simulink model "chap1_7"  (Simulink 6.3)
settings: Solver=ode4  StartTime=0.0  StopTime=1.0  RelTol=1e-3
undefined symbols (not defined in the file or in its folder): chap1_7ctrl
settings Model: LastModifiedBy=Administrator  ExtModeTrigMode=oneshot  ExtModeArmWhenConnect=off  StrictBusMsg=None
settings DataIOCC: Decimation=100  LimitDataPoints=off  SaveOutput=off  SaveTime=off
settings OptimizationCC: BlockReduction=off  BooleanDataType=off
settings DebuggingCC: SolverPrmCheckMsg=none
settings HardwareCC: TargetUnknown=on

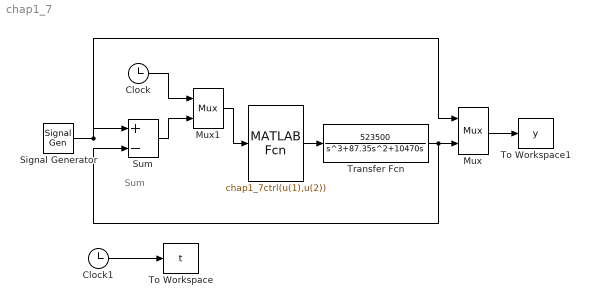
== system chap1_7 ==
  note: Sum
  "    " : MATLABFcn  MATLABFcn=chap1_7ctrl(u(1),u(2))
  Clock : Clock
      settings: Decimation=10
  Clock1 : Clock
      settings: Decimation=10
  Mux : Mux  Inputs=2
  Mux1 : Mux  Inputs=2
  Signal Generator : SignalGenerator  Amplitude=0.05
  Sum : Sum  Inputs=|+-  SaturateOnIntegerOverflow=on  InputSameDT=on
  To Workspace : ToWorkspace  VariableName=t  SampleTime=-1  SaveFormat=Array
  To Workspace1 : ToWorkspace  VariableName=y  SampleTime=-1  SaveFormat=Array
  Transfer Fcn : TransferFcn  Numerator=[523500]  Denominator=[1 87.35 10470 0]
  wires:
  Mux/1 -> To Workspace1/1
  Transfer Fcn/1 -> Sum/2, Mux/2
  Signal Generator/1 -> Sum/1, Mux/1
  Clock/1 -> Mux1/1
  Sum/1 -> Mux1/2
  Mux1/1 -> "    "/1
  "    "/1 -> Transfer Fcn/1
  Clock1/1 -> To Workspace/1
